simulink model "fsm_model"  (Simulink 8.0)
settings: Solver=ode3  StartTime=0.0  StopTime=inf  FixedStep=0.1  RelTol=1e-3
settings Model: Creator=caster  LastModifiedBy=davidrb
settings OptimizationCC: InlineParams=on  SimCompilerOptimization=On

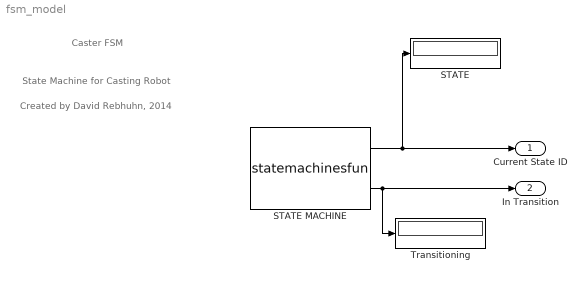
== system fsm_model ==
  note: State Machine for Casting Robot
  note: Caster FSM
  note: Created by David Rebhuhn, 2014
  STATE : Display
  STATE MACHINE : M-S-Function  FunctionName=statemachinesfun
      mask Display:
      | port_label('output',1,'Current State ID');
      | port_label('output',2,'In Transition');
  Transitioning : Display
  Current State ID : Outport
  In Transition : Outport  Port=2
  wires:
  STATE MACHINE/1 -> Current State ID/1, STATE/1
  STATE MACHINE/2 -> In Transition/1, Transitioning/1
